simulink model "APID_RLS2"  (R2021b)
settings: Solver=FixedStepAuto  StartTime=0.0  StopTime=6000  FixedStep=0.2  RelTol=1e-3  EnableMultiTasking=on
settings Model: SimulationMode=accelerator  Creator=issme  LastModifiedBy=ismt
settings SolverCC: AlgebraicLoopSolver=TrustRegion
settings DataIOCC: SaveFormat=Array  SignalLoggingSaveFormat=ModelDataLogs  ReturnWorkspaceOutputs=off  OutputSaveName=yout_RLS
settings OptimizationCC: ExpressionDepthLimit=2147483647  InitFltsAndDblsToZero=on  LifeSpan=inf
settings DebuggingCC: UnderspecifiedInitializationDetection=Classic  MergeDetectMultiDrivingBlocksExec=none  SolverPrmCheckMsg=warning  FcnCallInpInsideContextMsg=warning  StateNameClashWarn=warning  SFUnexpectedBacktrackingDiag=warning  SFNoUnconditionalDefaultTransitionDiag=warning  SFExecutionAtInitializationDiag=none  SFMachineParentedDataDiag=warning  ArithmeticOperatorsInVariantConditions=warning
settings HardwareCC: ProdBitPerPointer=32  ProdBitPerSizeT=32  ProdBitPerPtrDiffT=32  ProdLargestAtomicFloat=None  ProdIntDivRoundTo=Undefined  ProdEndianess=Unspecified  ProdWordSize=32  ProdHWDeviceType=32-bit Generic
settings ModelReferenceCC: PropagateSignalLabelsOutOfModel=off
settings CodeAppCC: StateflowObjectComments=on
settings GRTTargetCC: TargetLangStandard=C89/C90 (ANSI)  CombineOutputUpdateFcns=off  GRTInterface=on
settings ConfigComp: CovMetricSettings=dw  CovSaveCumulativeToWorkspaceVar=on  CovSaveSingleToWorkspaceVar=on

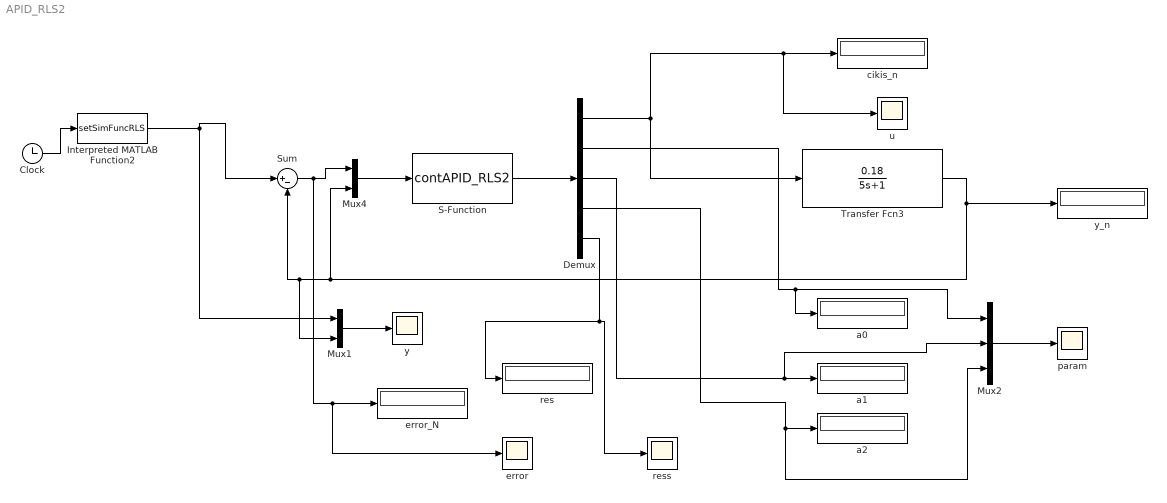
== system APID_RLS2 ==
  Clock : Clock
  Demux : Demux  Outputs=5
  Interpreted MATLAB Function2 : MATLABFcn  MATLABFcn=setSimFuncRLS
  Mux1 : Mux  Inputs=2
  Mux2 : Mux  Inputs=3
  Mux4 : Mux  Inputs=2
  S-Function : S-Function  FunctionName=contAPID_RLS2  SFunctionDeploymentMode=off  EnableBusSupport=off
  Sum : Sum  Inputs=|+-
  Transfer Fcn3 : TransferFcn  Numerator=[0.18]  Denominator=[5 1]
  a0 : Display
  a1 : Display
  a2 : Display
  cikis_n : Display
  error : Scope
  error_N : Display
  param : Scope
  res : Display
  ress : Scope
  u : Scope
  y : Scope
  y_n : Display
  wires:
  S-Function/1 -> Demux/1
  Interpreted MATLAB Function2/1 -> Sum/1, Mux1/1
  Transfer Fcn3/1 -> y_n/1, Mux4/2, Mux1/2, Sum/2
  Mux4/1 -> S-Function/1
  Sum/1 -> error/1, error_N/1, Mux4/1
  Demux/1 -> Transfer Fcn3/1, u/1, cikis_n/1
  Demux/2 -> a0/1, Mux2/1
  Demux/3 -> Mux2/2, a1/1
  Demux/4 -> Mux2/3, a2/1
  Mux1/1 -> y/1
  Mux2/1 -> param/1
  Demux/5 -> res/1, ress/1
  Clock/1 -> Interpreted MATLAB Function2/1
